simulink model "lab3_model"  (R2013b)
settings: Solver=ode3  StartTime=0.0  StopTime=10.0  FixedStep=0.01  RelTol=1e-3
libraries: fuzblock x1
settings Model: Creator=Vlad  LastModifiedBy=Vlad

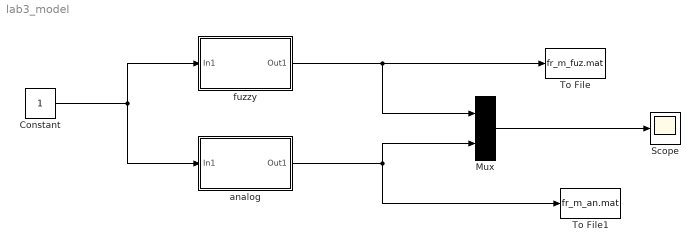
== system lab3_model ==
  Constant : Constant
  Mux : Mux  Inputs=2
  Scope : Scope
  To File : ToFile  Filename=fr_m_fuz.mat  MatrixName=fr_m_fuz
  To File1 : ToFile  Filename=fr_m_an.mat  MatrixName=fr_m_an
  analog : Subsystem
  fuzzy : Subsystem
  wires:
  Constant/1 -> fuzzy/1(In1), analog/1(In1)
  fuzzy/1(Out1) -> To File/1, Mux/1
  analog/1(Out1) -> Mux/2, To File1/1
  Mux/1 -> Scope/1

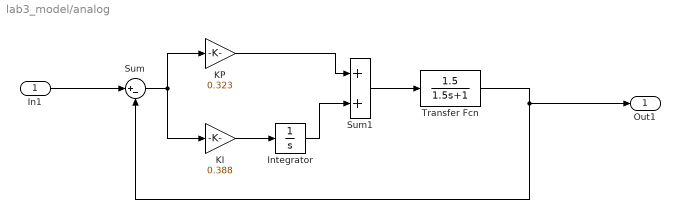
== system lab3_model/analog ==
  In1 : Inport
  Integrator : Integrator
  KI : Gain  Gain=0.388
  KP : Gain  Gain=0.323
  Sum : Sum  Inputs=|+-
  Sum1 : Sum  Inputs=|++
  Transfer Fcn : TransferFcn  Numerator=[1.5]  Denominator=[1.5 1]
  Out1 : Outport
  wires:
  Sum1/1 -> Transfer Fcn/1
  Sum/1 -> KP/1, KI/1
  Integrator/1 -> Sum1/2
  Transfer Fcn/1 -> Out1/1, Sum/2
  In1/1 -> Sum/1
  KP/1 -> Sum1/1
  KI/1 -> Integrator/1

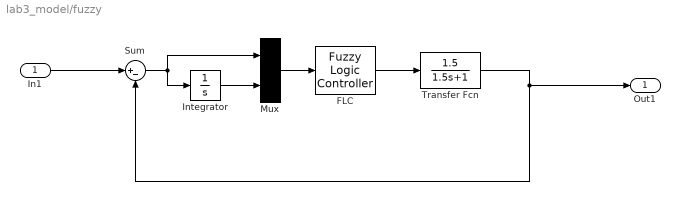
== system lab3_model/fuzzy ==
  In1 : Inport
  FLC : fuzblock/Fuzzy Logic  Controller  fis='lab3_fis.fis'
  Integrator : Integrator
  Mux : Mux  Inputs=2
  Sum : Sum  Inputs=|+-
  Transfer Fcn : TransferFcn  Numerator=[1.5]  Denominator=[1.5 1]
  Out1 : Outport
  wires:
  Mux/1 -> FLC/1
  FLC/1 -> Transfer Fcn/1
  Sum/1 -> Integrator/1, Mux/1
  Integrator/1 -> Mux/2
  Transfer Fcn/1 -> Out1/1, Sum/2
  In1/1 -> Sum/1
